simulink model "grading"  (R2021a)
settings: Solver=FixedStepDiscrete  StartTime=0.0  StopTime=10.0  RelTol=1e-3
settings Model: Creator=LEGION  LastModifiedBy=LEGION
settings OptimizationCC: DefaultParameterBehavior=Inlined  EnhancedBackFolding=on  PassReuseOutputArgsAs=Individual arguments  ZeroExternalMemoryAtStartup=off  ZeroInternalMemoryAtStartup=off  OptimizeBlockOrder=speed  DifferentSizesBufferReuse=on  OptimizationCustomize=off  EfficientTunableParamExpr=on
settings DebuggingCC: ParameterTunabilityLossMsg=error
settings SFSimCC: MATLABDynamicMemAlloc=off
settings RTWCC: SystemTargetFile=ert.tlc  GenCodeOnly=on  TemplateMakefile=ert_default_tmf  GenerateReport=on  IncludeHyperlinkInReport=on  LaunchReport=on  GenerateTraceInfo=on
settings CodeAppCC: ForceParamTrailComments=on  IgnoreCustomStorageClasses=off  OperatorAnnotations=on  SimulinkDataObjDesc=on  SFDataObjDesc=on  InsertBlockDesc=on
settings ERTTargetCC: TargetLangStandard=C99 (ISO)  GenerateSampleERTMain=on  InlinedParameterPlacement=NonHierarchical  ERTCustomFileTemplate=example_file_process.tlc  EnableUserReplacementTypes=on

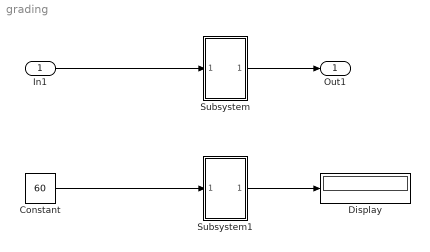
== system grading ==
  In1 : Inport
  Constant : Constant  Value=60
  Display : Display
  Subsystem : Subsystem
  Subsystem1 : Subsystem
  Out1 : Outport
  wires:
  In1/1 -> Subsystem/1(In1)
  Subsystem/1(Out1) -> Out1/1
  Constant/1 -> Subsystem1/1(In1)
  Subsystem1/1(Out1) -> Display/1

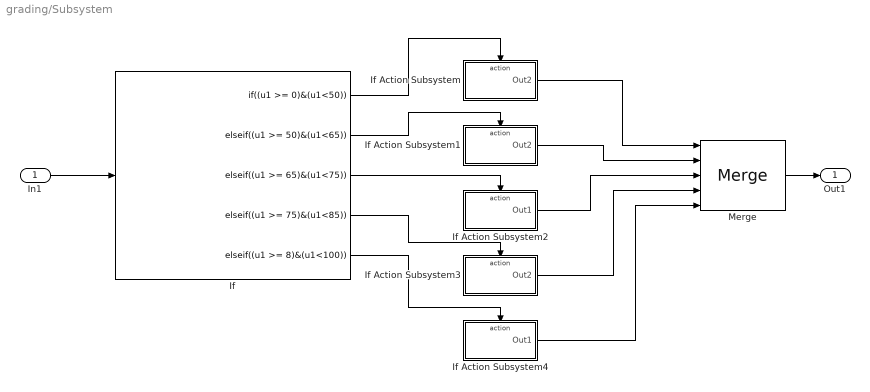
== system grading/Subsystem ==
  In1 : Inport
  If : If  IfExpression=(u1 >= 0)&(u1<50)  ElseIfExpressions=(u1 >= 50)&(u1<65),(u1 >= 65)&(u1<75),(u1 >= 75)&(u1<85),(u1 >= 8)&(u1<100)  ShowElse=off
  If Action Subsystem : Subsystem  TreatAsAtomicUnit=on
  If Action Subsystem1 : Subsystem  TreatAsAtomicUnit=on
  If Action Subsystem2 : Subsystem  TreatAsAtomicUnit=on
  If Action Subsystem3 : Subsystem  TreatAsAtomicUnit=on
  If Action Subsystem4 : Subsystem  TreatAsAtomicUnit=on
  Merge : Merge  Inputs=5
  Out1 : Outport
  wires:
  If/4 -> If Action Subsystem3/Action
  If Action Subsystem4/1(Out1) -> Merge/5
  If Action Subsystem1/1(Out2) -> Merge/2
  If/2 -> If Action Subsystem1/Action
  If Action Subsystem/1(Out2) -> Merge/1
  Merge/1 -> Out1/1
  If Action Subsystem3/1(Out2) -> Merge/4
  If Action Subsystem2/1(Out1) -> Merge/3
  If/5 -> If Action Subsystem4/Action
  If/3 -> If Action Subsystem2/Action
  If/1 -> If Action Subsystem/Action
  In1/1 -> If/1

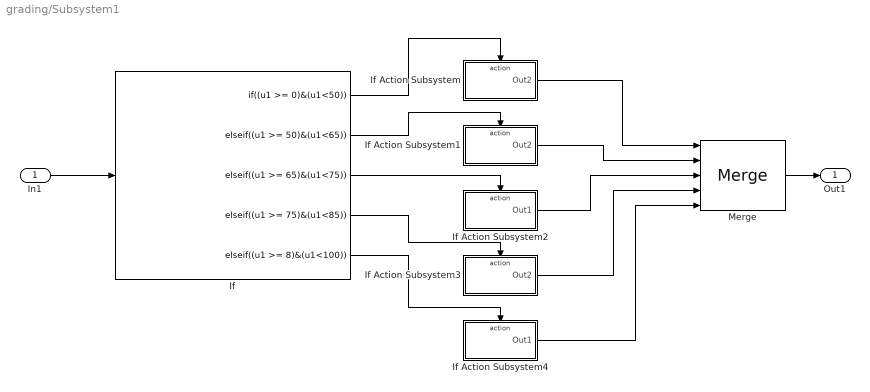
== system grading/Subsystem1 ==
  In1 : Inport
  If : If  IfExpression=(u1 >= 0)&(u1<50)  ElseIfExpressions=(u1 >= 50)&(u1<65),(u1 >= 65)&(u1<75),(u1 >= 75)&(u1<85),(u1 >= 8)&(u1<100)  ShowElse=off
  If Action Subsystem : Subsystem  TreatAsAtomicUnit=on
  If Action Subsystem1 : Subsystem  TreatAsAtomicUnit=on
  If Action Subsystem2 : Subsystem  TreatAsAtomicUnit=on
  If Action Subsystem3 : Subsystem  TreatAsAtomicUnit=on
  If Action Subsystem4 : Subsystem  TreatAsAtomicUnit=on
  Merge : Merge  Inputs=5
  Out1 : Outport
  wires:
  If/4 -> If Action Subsystem3/Action
  If Action Subsystem4/1(Out1) -> Merge/5
  If Action Subsystem1/1(Out2) -> Merge/2
  If/2 -> If Action Subsystem1/Action
  If Action Subsystem/1(Out2) -> Merge/1
  Merge/1 -> Out1/1
  If Action Subsystem3/1(Out2) -> Merge/4
  If Action Subsystem2/1(Out1) -> Merge/3
  If/5 -> If Action Subsystem4/Action
  If/3 -> If Action Subsystem2/Action
  If/1 -> If Action Subsystem/Action
  In1/1 -> If/1

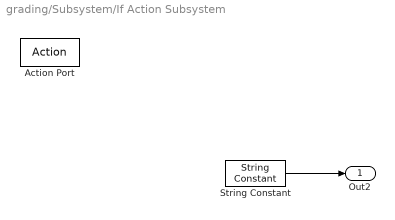
== system grading/Subsystem/If Action Subsystem ==
  Action Port : ActionPort  ActionPortLabel=if((u1 >= 0)&(u1<50))
  String Constant : StringConstant  String="\"Fail\""
  Out2 : Outport
  wires:
  String Constant/1 -> Out2/1

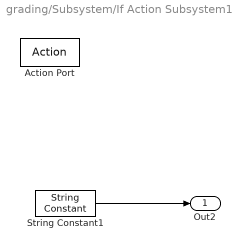
== system grading/Subsystem/If Action Subsystem1 ==
  Action Port : ActionPort  ActionPortLabel=elseif((u1 >= 50)&(u1<65))
  String Constant1 : StringConstant  String="\"Pass\""
  Out2 : Outport
  wires:
  String Constant1/1 -> Out2/1

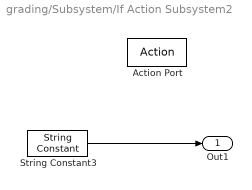
== system grading/Subsystem/If Action Subsystem2 ==
  Action Port : ActionPort  ActionPortLabel=elseif((u1 >= 65)&(u1<75))
  String Constant3 : StringConstant  String="\" Good\""
  Out1 : Outport
  wires:
  String Constant3/1 -> Out1/1

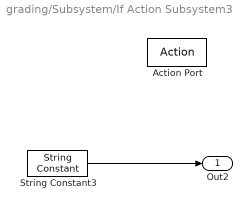
== system grading/Subsystem/If Action Subsystem3 ==
  Action Port : ActionPort  ActionPortLabel=elseif((u1 >= 75)&(u1<85))
  String Constant3 : StringConstant  String="\"Very Good\""
  Out2 : Outport
  wires:
  String Constant3/1 -> Out2/1

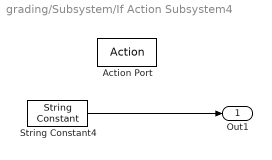
== system grading/Subsystem/If Action Subsystem4 ==
  Action Port : ActionPort  ActionPortLabel=elseif((u1 >= 8)&(u1<100))
  String Constant4 : StringConstant  String="\"Excellent\""
  Out1 : Outport
  wires:
  String Constant4/1 -> Out1/1

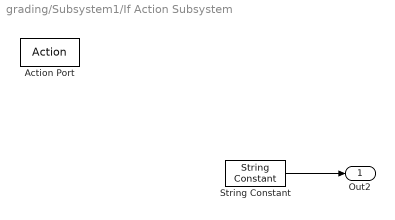
== system grading/Subsystem1/If Action Subsystem ==
  Action Port : ActionPort  ActionPortLabel=if((u1 >= 0)&(u1<50))
  String Constant : StringConstant  String="\"Fail\""
  Out2 : Outport
  wires:
  String Constant/1 -> Out2/1

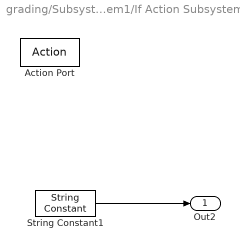
== system grading/Subsystem1/If Action Subsystem1 ==
  Action Port : ActionPort  ActionPortLabel=elseif((u1 >= 50)&(u1<65))
  String Constant1 : StringConstant  String="\"Pass\""
  Out2 : Outport
  wires:
  String Constant1/1 -> Out2/1

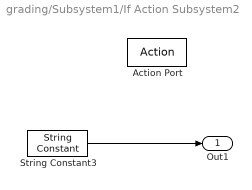
== system grading/Subsystem1/If Action Subsystem2 ==
  Action Port : ActionPort  ActionPortLabel=elseif((u1 >= 65)&(u1<75))
  String Constant3 : StringConstant  String="\" Good\""
  Out1 : Outport
  wires:
  String Constant3/1 -> Out1/1

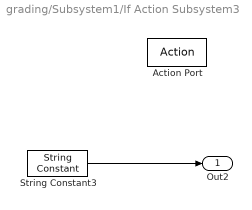
== system grading/Subsystem1/If Action Subsystem3 ==
  Action Port : ActionPort  ActionPortLabel=elseif((u1 >= 75)&(u1<85))
  String Constant3 : StringConstant  String="\"Very Good\""
  Out2 : Outport
  wires:
  String Constant3/1 -> Out2/1

== system grading/Subsystem1/If Action Subsystem4 ==
  Action Port : ActionPort  ActionPortLabel=elseif((u1 >= 8)&(u1<100))
  String Constant4 : StringConstant  String="\"Excellent\""
  Out1 : Outport
  wires:
  String Constant4/1 -> Out1/1
